simulink model "MODELODETURBINADERIOV3"  (R2017b)
settings: Solver=FixedStepAuto  StartTime=0.0  StopTime=200  FixedStep=50e-3  RelTol=1e-3
values from neighbouring files (symbols this model uses):
  A = pi()*((D/2)^2)    [MODELOHIDRO.m]    (also in MODELOHIDROV10.m; MODELOHIDROV2.m; MODELOHIDROV3.m; MODELOHIDROV4.m)
  B = 0    [MODELOHIDRO.m]    (also in MODELOHIDROV10.m; MODELOHIDROV2.m; MODELOHIDROV3.m; MODELOHIDROV4.m)
  beta = 0    [MODELOHIDRO.m]    (also in MODELOHIDROV10.m; MODELOHIDROV2.m; MODELOHIDROV3.m; MODELOHIDROV4.m)
  Bi = 0.2287    [MODELOHIDRO.m]    (also in MODELOHIDROV10.m = 0.1; MODELOHIDROV2.m; MODELOHIDROV3.m; MODELOHIDROV4.m = 0.005)
  den = 1000    [MODELOHIDRO.m]    (also in MODELOHIDROV10.m; MODELOHIDROV2.m; MODELOHIDROV3.m; MODELOHIDROV4.m)
  J = 16.1919e-4    (= 0.00161919)    [MODELOHIDROV10.m]    (also in MODELOHIDROV2.m = 100; MODELOHIDROV3.m = 10; MODELOHIDROV4.m; MODELOHIDROV7.m)
  Ji = 1    [MODELOHIDRO.m]    (also in MODELOHIDROV10.m = 1.72; MODELOHIDROV2.m; MODELOHIDROV3.m; MODELOHIDROV4.m = 0.0465)
  k = 1    [MODELOHIDRO.m]    (also in MODELOHIDROV2.m; MODELOHIDROV3.m)
  Kb = 1.8    [MODELOHIDRO.m]    (also in MODELOHIDROV10.m = 6.2; MODELOHIDROV2.m; MODELOHIDROV3.m; MODELOHIDROV4.m = 0.027)
  Kp = 0.4    [MODELOHIDRO.m]    (also in MODELOHIDROV10.m = 5.6627; MODELOHIDROV2.m; MODELOHIDROV3.m; MODELOHIDROV4.m = 0.027)
  L_d = 38e-3    (= 0.038)    [MODELOHIDROV2.m]    (also in MODELOHIDROV3.m; MODELOHIDROV4.m; MODELOHIDROV7.m)
  L_q = 9.03e-3    (= 0.00903)    [MODELOHIDROV2.m]    (also in MODELOHIDROV3.m; MODELOHIDROV4.m; MODELOHIDROV7.m)
  Lambda = 0.48    [MODELOHIDROV2.m]    (also in MODELOHIDROV3.m; MODELOHIDROV4.m; MODELOHIDROV7.m)
  m = 5    [MODELOHIDRO.m]    (also in MODELOHIDROV2.m; MODELOHIDROV3.m)
  P = 1    [MODELOHIDROV2.m]    (also in MODELOHIDROV3.m; MODELOHIDROV4.m; MODELOHIDROV7.m)
  r = D/2    (= 0.5)    [MODELOHIDRO.m]    (also in MODELOHIDROV10.m; MODELOHIDROV2.m; MODELOHIDROV3.m; MODELOHIDROV4.m)
  Ri = 0.6    [MODELOHIDRO.m]    (also in MODELOHIDROV10.m = 0.973; MODELOHIDROV2.m; MODELOHIDROV3.m; MODELOHIDROV4.m = 1)
  Rs = 1.649    [MODELOHIDROV2.m]    (also in MODELOHIDROV3.m; MODELOHIDROV4.m; MODELOHIDROV7.m)
  T_d = 0    [MODELOHIDRO.m]    (also in MODELOHIDROV10.m; MODELOHIDROV2.m; MODELOHIDROV3.m; MODELOHIDROV4.m)
  z = 2    [MODELOHIDRO.m]    (also in MODELOHIDROV2.m; MODELOHIDROV3.m)
undefined symbols (not defined in the file or in its folder): sigbuilder_block
libraries: simulink x1
settings Model: Creator=zni.uao  LastModifiedBy=Hp 14
settings CodeAppCC: StateflowObjectComments=on
settings SimscapeCC: SimscapeNormalizeSystem=off

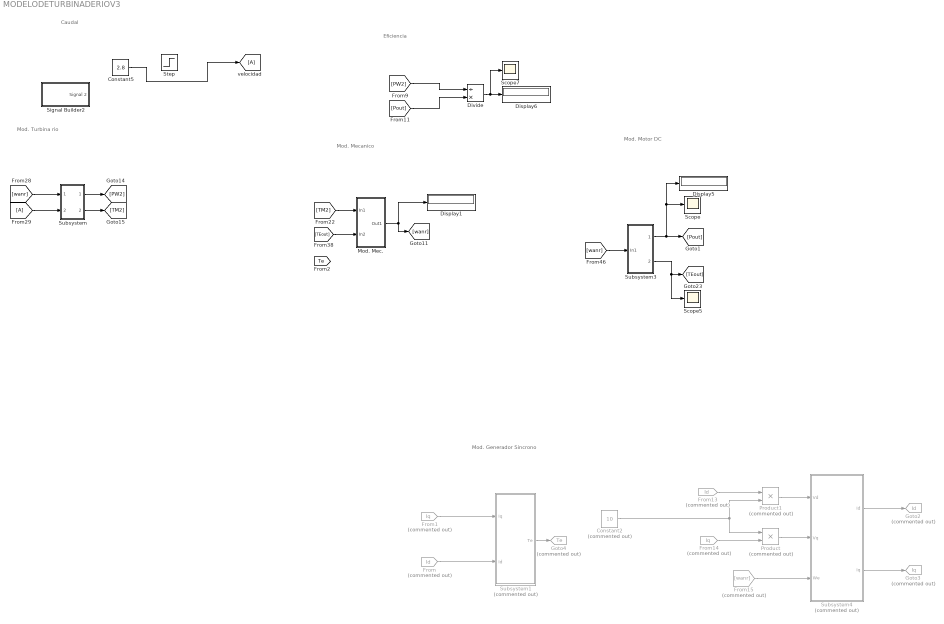
== system MODELODETURBINADERIOV3 ==
  note: Mod. Motor DC
  note: Mod. Turbina rio
  note: Mod. Mecanico
  note: Mod. Generador Sincrono
  note: Eficiencia
  note: Caudal
  Constant2 : Constant  Commented=on  Value=10
  Constant5 : Constant  Value=2.8
  Display1 : Display
  Display5 : Display
  Display6 : Display
  Divide : Product  Inputs=/*
  From : From  Commented=on  GotoTag=Id  TagVisibility=global
  From1 : From  Commented=on  GotoTag=Iq  TagVisibility=global
  From13 : From  Commented=on  GotoTag=Id  TagVisibility=global
  From14 : From  Commented=on  GotoTag=Iq  TagVisibility=global
  From15 : From  Commented=on  GotoTag=wanr
  Goto2 : Goto  Commented=on  GotoTag=Id  TagVisibility=global
  Goto3 : Goto  Commented=on  GotoTag=Iq  TagVisibility=global
  Goto4 : Goto  Commented=on  GotoTag=Te  TagVisibility=global
  Mod. Mec. : Subsystem
  Product : Product  Commented=on
  Product1 : Product  Commented=on
  Scope : Scope
  Scope5 : Scope
  Scope7 : Scope
  Signal Builder2 : Subsystem  Tag=STV Subsys  LoadFcn=sigbuilder_block('load');  StartFcn=sigbuilder_block('start');  StopFcn=sigbuilder_block('stop');  ClipboardFcn=sigbuilder_block('clipboard');  mask(Sigbuilder block){tuvar=[0:10]}
      mask help: Simulink:masks:SigbuilderBlock_MD
      mask init:
      | if ~strcmp(get_param(bdroot(gcbh),'SimulationStatus'),'stopped') tuvar = sigbuilder_block('maskInit'); end
      settings: CopyFcn=sigbuilder_block('copy');  DeleteFcn=sigbuilder_block('delete');  ModelCloseFcn=sigbuilder_block('modelClose');  PreSaveFcn=sigbuilder_block('preSave');  PauseFcn=sigbuilder_block('pause');  ContinueFcn=sigbuilder_block('continue');  NameChangeFcn=sigbuilder_block('namechange');  OpenFcn=sigbuilder_block('open',[197.25 66 550.5 359.25 ]);  CloseFcn=sigbuilder_block('close');
      mask Display: plot(0, 0, 100, 100,[2, 2, 32, 32, 2], [68, 8, 8, 68, 68],[32, 2], [38, 38], [32, 19, 2],[53, 60, 44], [32, 17, 17, 2],[16, 16, 31, 31]);txt = getActiveGroup(gcbh);text(2, 100, txt,'verticalAlignment', 'top');
  Step : Step  Time=10  Before=2.5  After=2.888  SampleTime=0
  Subsystem : Subsystem
  Subsystem1 : Subsystem  Commented=on
  Subsystem3 : Subsystem
  Subsystem4 : Subsystem  Commented=on
  wires:
  [PW2] -> Divide/1
  [Pout] -> Divide/2
  Divide/1 -> Scope7/1, Display6/1
  Subsystem4/1(Id) -> Goto2/1
  From13/1 -> Product1/1
  From14/1 -> Product/2
  Constant2/1 -> Product/1, Product1/2
  Product/1 -> Subsystem4/2(Vq)
  Product1/1 -> Subsystem4/1(Vd)
  Subsystem4/2(Iq) -> Goto3/1
  From15/1 -> Subsystem4/3(We)
  [wanr] -> Subsystem/1(In1)
  [A] -> Subsystem/2(In2)
  Subsystem/1(Out1) -> [PW2]
  Subsystem/2(Out2) -> [TM2]
  Mod. Mec./1(Out1) -> [wanr], Display1/1
  [TM2] -> Mod. Mec./1(In1)
  Subsystem3/1(Out1) -> Display5/1, Scope/1, [Pout]
  Subsystem3/2(Out2) -> [TEout], Scope5/1
  [wanr] -> Subsystem3/1(In1)
  From/1 -> Subsystem1/2(Id)
  From1/1 -> Subsystem1/1(Iq)
  Subsystem1/1(Te) -> Goto4/1
  [TEout] -> Mod. Mec./2(In2)
  Constant5/1 -> [A]

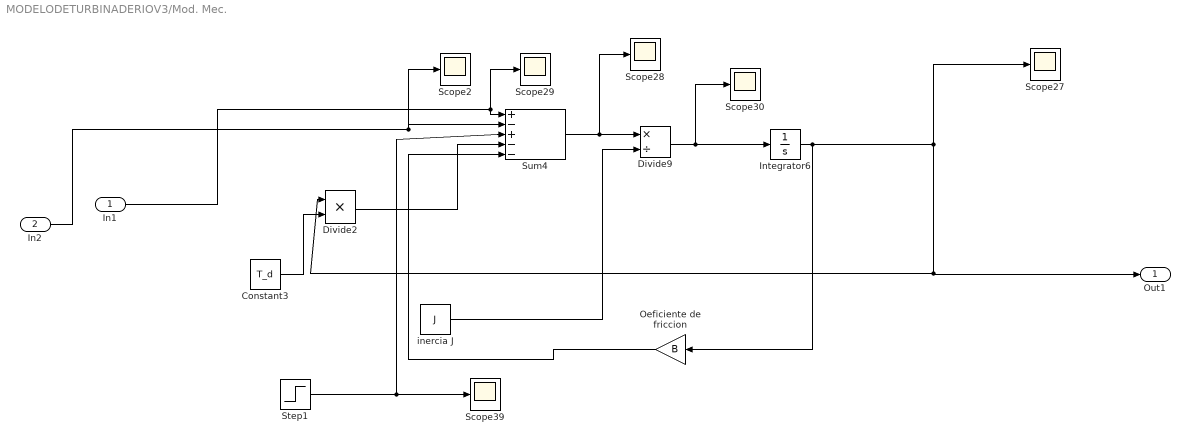
== system MODELODETURBINADERIOV3/Mod. Mec. ==
  In1 : Inport
  In2 : Inport  Port=2
  Constant3 : Constant  Value=T_d
  Divide2 : Product  Inputs=**
  Divide9 : Product  Inputs=*/
  Integrator6 : Integrator  InitialCondition=10
  Oeficiente de friccion : Gain  Gain=B
  Scope{2,27..30,39} (6 alike) : Scope
  Step1 : Step  Time=3  Before=5  After=0  SampleTime=0
  Sum4 : Sum  Inputs=|+-+--
  inercia J : Constant  Value=J
  Out1 : Outport
  wires:
  inercia J/1 -> Divide9/2
  Constant3/1 -> Divide2/2
  Divide2/1 -> Sum4/4
  Oeficiente de friccion/1 -> Sum4/5
  Step1/1 -> Scope39/1, Sum4/3
  Sum4/1 -> Scope28/1, Divide9/1
  In1/1 -> Scope29/1, Sum4/1
  In2/1 -> Scope2/1, Sum4/2
  Divide9/1 -> Scope30/1, Integrator6/1
  Integrator6/1 -> Out1/1, Divide2/1, Scope27/1, Oeficiente de friccion/1

== system MODELODETURBINADERIOV3/Signal Builder2 ==
  Demux : Demux  Tag=STV Demux  Outputs=1
  FromWs : FromWorkspace  Tag=STV FromWs  VariableName=tuvar  SampleTime=0
      SigBuilderData=|
      | common.afterFinalStr = 'Extrapolate'
      | common.sampleTime = 0
      | dataSet.timeRange = [0 10]
      | dataSet.name = 'Group 1'
      | sbobj.Groups.Name = 'Group 1'
      | sbobj.Groups.Signals.Name = 'Signal 2'
      | sbobj.Groups.Signals.XData = [0 3 3 5 5 10]
      | sbobj.Groups.Signals.YData = [2 2 2.5 2.5 2.8 2.8]
  Signal 2 : Outport  Tag=STV Outport
  wires:
  FromWs/1 -> Demux/1
  Demux/1 -> Signal 2/1

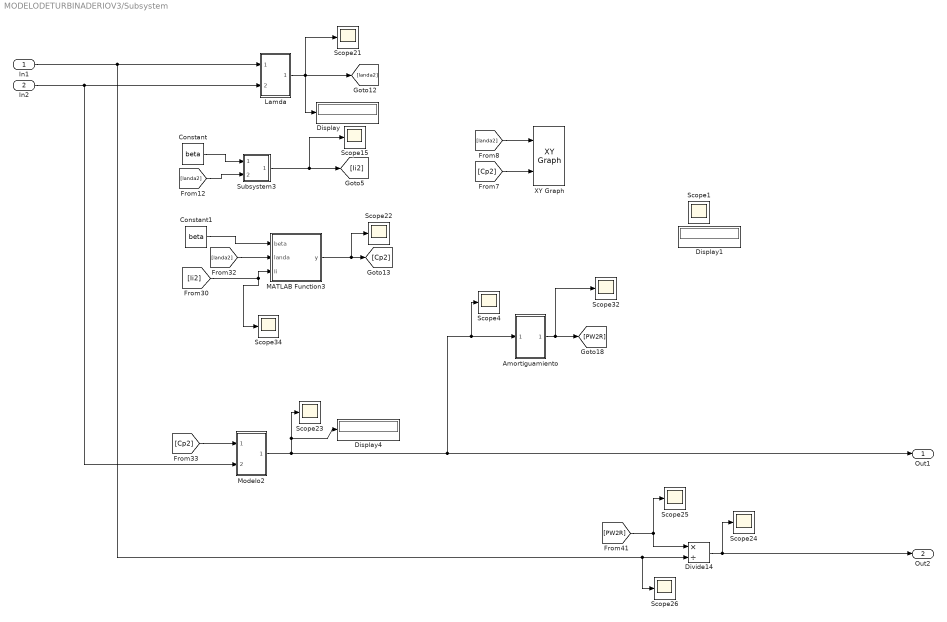
== system MODELODETURBINADERIOV3/Subsystem ==
  In1 : Inport
  In2 : Inport  Port=2
  Amortiguamiento : Subsystem
  Constant : Constant  Value=beta
  Constant1 : Constant  Value=beta
  Display : Display
  Display1 : Display
  Display4 : Display
  Divide14 : Product  Inputs=*/
  Lamda : Subsystem
  MATLAB Function3 : MATLAB Function  TreatAsAtomicUnit=on
  Modelo2 : Subsystem
  Scope{1,4,15,21..26,32,34} (11 alike) : Scope
  Subsystem3 : Subsystem
  XY Graph : simulink/Sinks/XY Graph  xmin=1  xmax=20  ymin=0  ymax=0.56  st=0.1
  Out1 : Outport
  Out2 : Outport  Port=2
  wires:
  Modelo2/1(Out1) -> Amortiguamiento/1(In1), Scope4/1, Out1/1, Display4/1, Scope23/1
  Constant1/1 -> MATLAB Function3/1(beta)
  Divide14/1 -> Out2/1, Scope24/1
  [Ii2] -> Scope34/1, MATLAB Function3/3(Ii)
  [Cp2] -> Modelo2/1(In1)
  [PW2R] -> Scope25/1, Divide14/1
  In1/1 -> Scope26/1, Divide14/2, Lamda/1(In1)
  [landa2] -> MATLAB Function3/2(landa)
  In2/1 -> Modelo2/2(In2), Lamda/2(In2)
  Lamda/1(Out1) -> Display/1, [landa2], Scope21/1
  MATLAB Function3/1(y) -> Scope22/1, [Cp2]
  [landa2] -> XY Graph/1
  Constant/1 -> Subsystem3/1(In1)
  [landa2] -> Subsystem3/2(In2)
  Amortiguamiento/1(Out1) -> Scope32/1, [PW2R]
  Subsystem3/1(Out1) -> Scope15/1, [Ii2]
  [Cp2] -> XY Graph/2

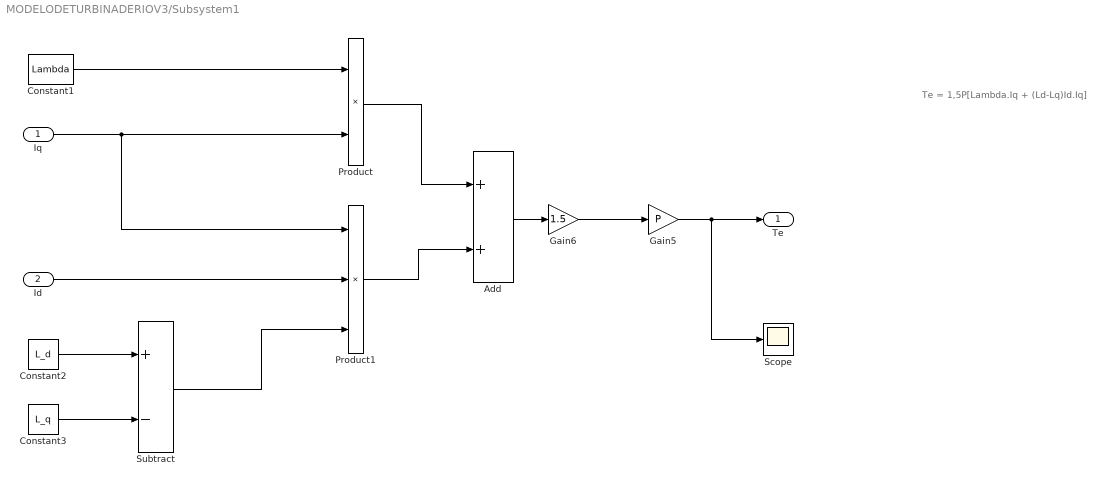
== system MODELODETURBINADERIOV3/Subsystem1 ==
  note: Te = 1,5P[Lambda.Iq + (Ld-Lq)Id.Iq]
  Iq : Inport
  Id : Inport  Port=2
  Add : Sum
  Constant1 : Constant  Value=Lambda
  Constant2 : Constant  Value=L_d
  Constant3 : Constant  Value=L_q
  Gain5 : Gain  Gain=P
  Gain6 : Gain  Gain=1.5
  Product : Product
  Product1 : Product  Inputs=3
  Scope : Scope
  Subtract : Sum  Inputs=+-
  Te : Outport
  wires:
  Product1/1 -> Add/2
  Iq/1 -> Product1/1, Product/2
  Constant1/1 -> Product/1
  Gain5/1 -> Scope/1, Te/1
  Subtract/1 -> Product1/3
  Id/1 -> Product1/2
  Gain6/1 -> Gain5/1
  Add/1 -> Gain6/1
  Product/1 -> Add/1
  Constant2/1 -> Subtract/1
  Constant3/1 -> Subtract/2

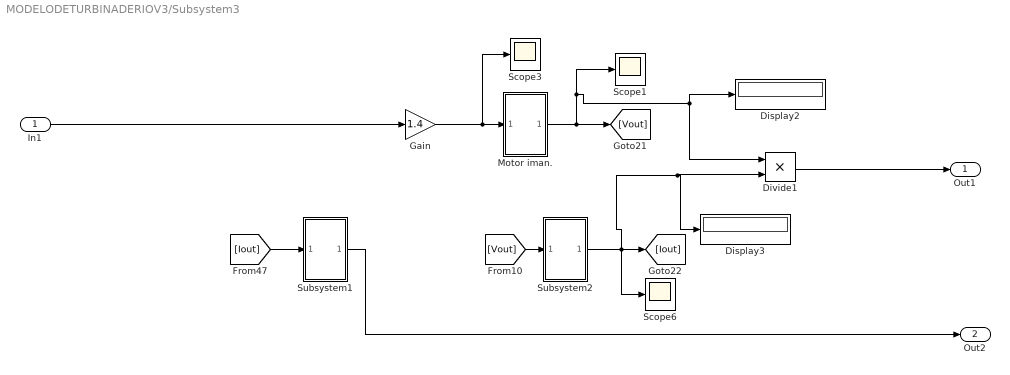
== system MODELODETURBINADERIOV3/Subsystem3 ==
  In1 : Inport
  Display2 : Display
  Display3 : Display
  Divide1 : Product  Inputs=**
  Gain : Gain  Gain=1.4
  Motor iman. : Subsystem
  Scope1 : Scope
  Scope3 : Scope
  Scope6 : Scope
  Subsystem1 : Subsystem
  Subsystem2 : Subsystem
  Out1 : Outport
  Out2 : Outport  Port=2
  wires:
  Motor iman./1(Out1) -> Divide1/1, Display2/1, Scope1/1, [Vout]
  Subsystem1/1(Out1) -> Out2/1
  [Iout] -> Subsystem1/1(In1)
  Subsystem2/1(Out1) -> Divide1/2, Display3/1, Scope6/1, [Iout]
  Divide1/1 -> Out1/1
  Gain/1 -> Scope3/1, Motor iman./1(In1)
  In1/1 -> Gain/1
  [Vout] -> Subsystem2/1(In1)

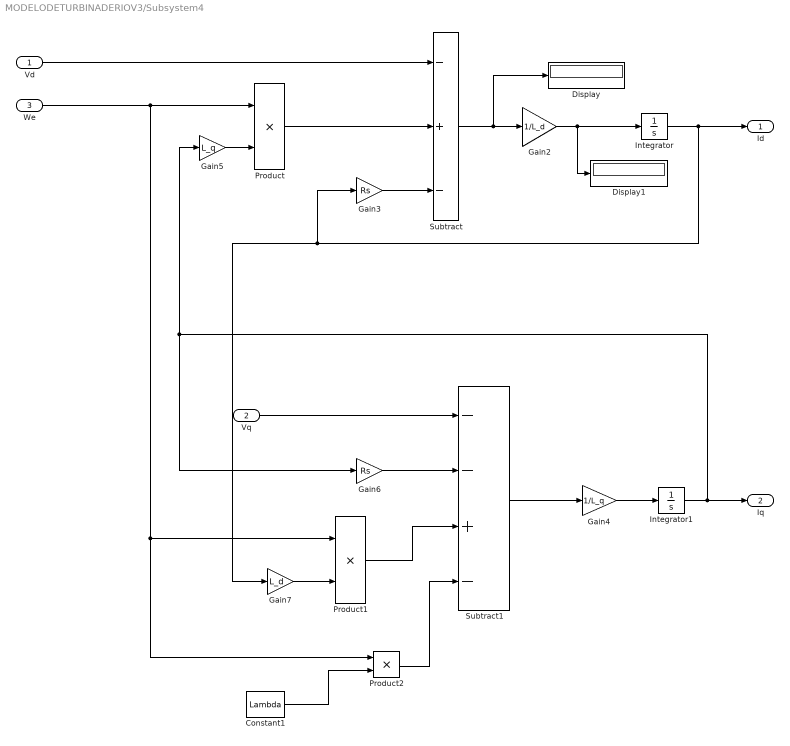
== system MODELODETURBINADERIOV3/Subsystem4 ==
  Vd : Inport
  Vq : Inport  Port=2
  We : Inport  Port=3
  Constant1 : Constant  Value=Lambda
  Display : Display
  Display1 : Display
  Gain2 : Gain  Gain=1/L_d
  Gain3 : Gain  Gain=Rs
  Gain4 : Gain  Gain=1/L_q
  Gain5 : Gain  Gain=L_q
  Gain6 : Gain  Gain=Rs
  Gain7 : Gain  Gain=L_d
  Integrator : Integrator
  Integrator1 : Integrator
  Product : Product
  Product1 : Product
  Product2 : Product
  Subtract : Sum  Inputs=-+-
  Subtract1 : Sum  Inputs=--+-
  Id : Outport
  Iq : Outport  Port=2
  wires:
  Integrator1/1 -> Gain6/1, Gain5/1, Iq/1
  We/1 -> Product/1, Product2/1, Product1/1
  Product1/1 -> Subtract1/3
  Gain7/1 -> Product1/2
  Product/1 -> Subtract/2
  Integrator/1 -> Id/1, Gain7/1, Gain3/1
  Gain4/1 -> Integrator1/1
  Gain2/1 -> Display1/1, Integrator/1
  Gain5/1 -> Product/2
  Subtract/1 -> Display/1, Gain2/1
  Subtract1/1 -> Gain4/1
  Vq/1 -> Subtract1/1
  Gain6/1 -> Subtract1/2
  Vd/1 -> Subtract/1
  Constant1/1 -> Product2/2
  Product2/1 -> Subtract1/4
  Gain3/1 -> Subtract/3

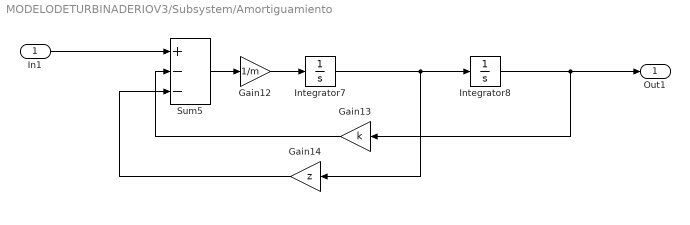
== system MODELODETURBINADERIOV3/Subsystem/Amortiguamiento ==
  In1 : Inport
  Gain12 : Gain  Gain=1/m
  Gain13 : Gain  Gain=k
  Gain14 : Gain  Gain=z
  Integrator7 : Integrator
  Integrator8 : Integrator
  Sum5 : Sum  Inputs=+--
  Out1 : Outport
  wires:
  Gain13/1 -> Sum5/2
  Integrator8/1 -> Out1/1, Gain13/1
  Integrator7/1 -> Gain14/1, Integrator8/1
  Sum5/1 -> Gain12/1
  Gain12/1 -> Integrator7/1
  Gain14/1 -> Sum5/3
  In1/1 -> Sum5/1

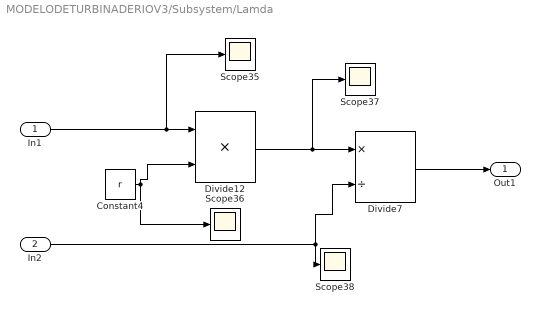
== system MODELODETURBINADERIOV3/Subsystem/Lamda ==
  In1 : Inport
  In2 : Inport  Port=2
  Constant4 : Constant  Value=r
  Divide12 : Product  Inputs=**
  Divide7 : Product  Inputs=*/
  Scope{35..38} (4 alike) : Scope
  Out1 : Outport
  wires:
  Divide7/1 -> Out1/1
  Constant4/1 -> Divide12/2, Scope36/1
  In2/1 -> Divide7/2, Scope38/1
  Divide12/1 -> Scope37/1, Divide7/1
  In1/1 -> Scope35/1, Divide12/1

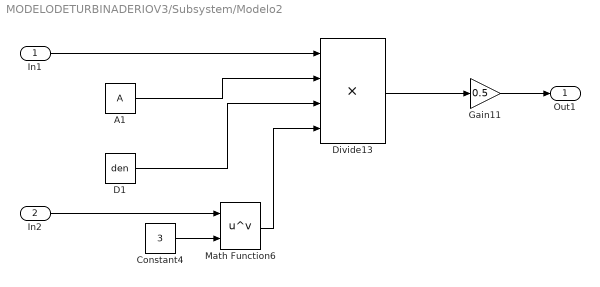
== system MODELODETURBINADERIOV3/Subsystem/Modelo2 ==
  In1 : Inport
  In2 : Inport  Port=2
  A1 : Constant  Value=A
  Constant4 : Constant  Value=3
  D1 : Constant  Value=den
  Divide13 : Product  Inputs=****  SaturateOnIntegerOverflow=on  RndMeth=Zero
  Gain11 : Gain  Gain=0.5
  Math Function6 : Math  Operator=pow  SaturateOnIntegerOverflow=on
  Out1 : Outport
  wires:
  Constant4/1 -> Math Function6/2
  Divide13/1 -> Gain11/1
  D1/1 -> Divide13/3
  In1/1 -> Divide13/1
  Gain11/1 -> Out1/1
  A1/1 -> Divide13/2
  In2/1 -> Math Function6/1
  Math Function6/1 -> Divide13/4

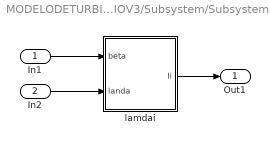
== system MODELODETURBINADERIOV3/Subsystem/Subsystem3 ==
  In1 : Inport
  In2 : Inport  Port=2
  lamdai : MATLAB Function  TreatAsAtomicUnit=on
  Out1 : Outport
  wires:
  lamdai/1(Ii) -> Out1/1
  In2/1 -> lamdai/2(landa)
  In1/1 -> lamdai/1(beta)

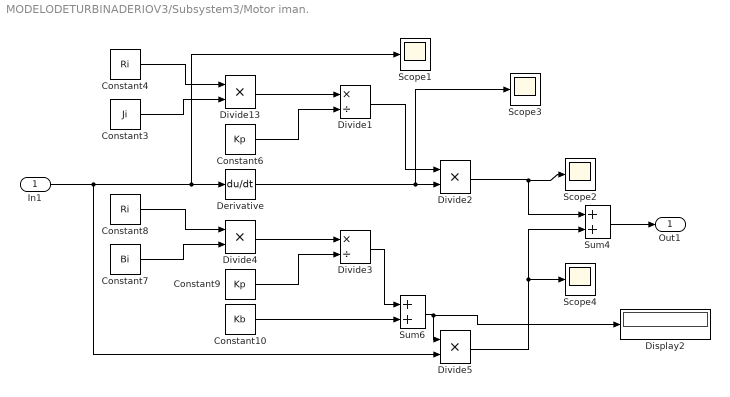
== system MODELODETURBINADERIOV3/Subsystem3/Motor iman. ==
  In1 : Inport
  Constant10 : Constant  Value=Kb
  Constant3 : Constant  Value=Ji
  Constant4 : Constant  Value=Ri
  Constant6 : Constant  Value=Kp
  Constant7 : Constant  Value=Bi
  Constant8 : Constant  Value=Ri
  Constant9 : Constant  Value=Kp
  Derivative : Derivative
  Display2 : Display
  Divide1 : Product  Inputs=*/  SaturateOnIntegerOverflow=on  RndMeth=Zero
  Divide{2,4..5,13} (4 alike) : Product  Inputs=**  SaturateOnIntegerOverflow=on  RndMeth=Zero
  Divide3 : Product  Inputs=*/  SaturateOnIntegerOverflow=on  RndMeth=Zero
  Scope{1..4} (4 alike) : Scope
  Sum4 : Sum
  Sum6 : Sum
  Out1 : Outport
  wires:
  Constant10/1 -> Sum6/2
  Divide2/1 -> Scope2/1, Sum4/1
  In1/1 -> Divide5/2, Scope1/1, Derivative/1
  Divide3/1 -> Sum6/1
  Divide13/1 -> Divide1/1
  Constant6/1 -> Divide1/2
  Constant4/1 -> Divide13/1
  Sum6/1 -> Display2/1, Divide5/1
  Divide1/1 -> Divide2/1
  Constant3/1 -> Divide13/2
  Constant9/1 -> Divide3/2
  Divide4/1 -> Divide3/1
  Constant7/1 -> Divide4/2
  Constant8/1 -> Divide4/1
  Derivative/1 -> Scope3/1, Divide2/2
  Sum4/1 -> Out1/1
  Divide5/1 -> Scope4/1, Sum4/2

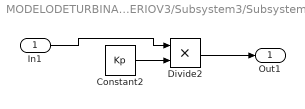
== system MODELODETURBINADERIOV3/Subsystem3/Subsystem1 ==
  In1 : Inport
  Constant2 : Constant  Value=Kp
  Divide2 : Product  Inputs=**
  Out1 : Outport
  wires:
  In1/1 -> Divide2/1
  Constant2/1 -> Divide2/2
  Divide2/1 -> Out1/1

== system MODELODETURBINADERIOV3/Subsystem3/Subsystem2 ==
  In1 : Inport
  Constant : Constant  Value=5
  Divide1 : Product  Inputs=*/
  Out1 : Outport
  wires:
  Divide1/1 -> Out1/1
  Constant/1 -> Divide1/2
  In1/1 -> Divide1/1

== matlab function MODELODETURBINADERIOV3/Subsystem/MATLAB Function3 ==
  data: beta input; y output; landa input; Ii input
function y = fcn(beta, landa,Ii)
w=0.5176; 
w1=116/Ii;
 w2=0.4*beta;
 w3=exp(-21/Ii);
 
 cp=w*(w1-w2-5)*w3+0.0068*landa;
 
 
 
 
 
y=cp;

== matlab function MODELODETURBINADERIOV3/Subsystem/Subsystem3/lamdai ==
  data: beta input; Ii output; landa input
function Ii = fcn(beta,landa)


Iii=(1/((landa+(0.08*beta))))-((0.035)/((beta^3)+1));
Ii=1/Iii;
